simulink library "Satellite_Dynamics_lib"  (R2018b)
settings: Solver=ode45  StartTime=0.0  StopTime=10.0  RelTol=1e-3  EnableMultiTasking=on
undefined symbols (not defined in the file or in its folder): simParams
libraries: dspinverses x1, vrlib x1
settings Model: Creator=devantormey  LastModifiedBy=devantormey
settings DataIOCC: LimitDataPoints=on
settings OptimizationCC: LifeSpan=inf
settings DebuggingCC: AllowSymbolicDim=off  SFUnexpectedBacktrackingDiag=warning  SFNoUnconditionalDefaultTransitionDiag=warning
settings SFSimCC: SimUseLocalCustomCode=off
settings RTWCC: RTWUseLocalCustomCode=off
settings CodeAppCC: StateflowObjectComments=on
settings GRTTargetCC: TargetLangStandard=C89/C90 (ANSI)  GeneratePreprocessorConditionals=Disable all
settings ConfigComp: CovMetricSettings=dw  CovHtmlReporting=on  CovSaveCumulativeToWorkspaceVar=on  CovSaveSingleToWorkspaceVar=on  CovExternalEMLEnable=off

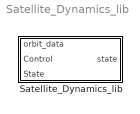
== system Satellite_Dynamics_lib ==
  Satellite_Dynamics_lib : Subsystem

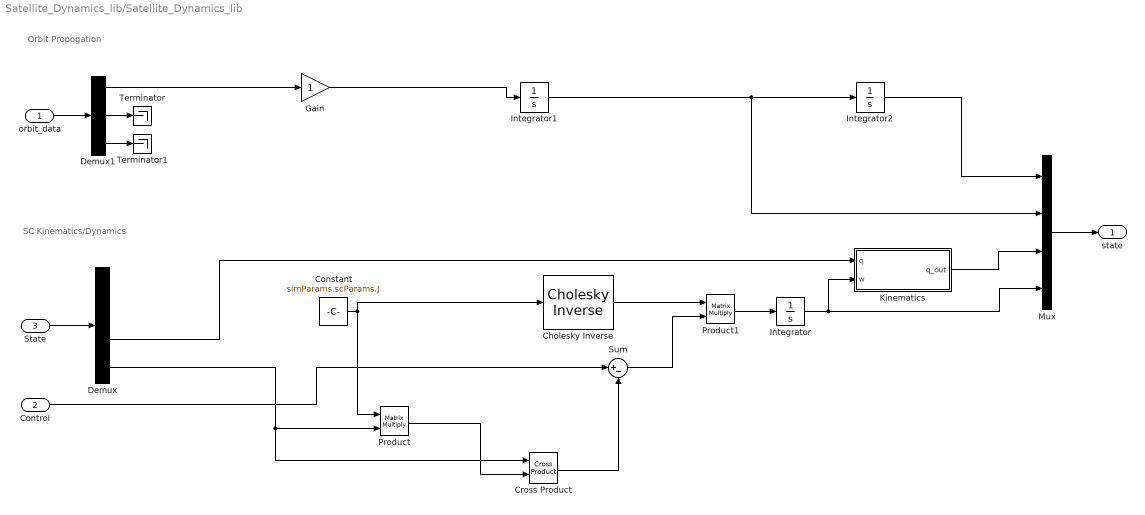
== system Satellite_Dynamics_lib/Satellite_Dynamics_lib ==
  note: Orbit Propogation
  note: SC Kinematics/Dynamics
  orbit_data : Inport
  Control : Inport  Port=2
  State : Inport  Port=3
  Cholesky Inverse : dspinverses/Cholesky Inverse  errmode=Warning
      settings: SourceProductName=DSP System Toolbox  SourceProductBaseCode=DS
  Constant : Constant  Value=simParams.scParams.J
  Cross Product : vrlib/Utilities/Cross Product
      settings: SourceProductBaseCode=VR
  Demux : Demux  Outputs=[3 3 4 3]
  Demux1 : Demux  Outputs=[3 3 1]
  Gain : Gain
  Integrator : Integrator  InitialCondition=simParams.initialConditions.w0
  Integrator1 : Integrator  InitialCondition=simParams.initialConditions.v0
  Integrator2 : Integrator  InitialCondition=simParams.initialConditions.r0
  Kinematics : Subsystem
  Mux : Mux  Inputs=[3 3 4 3]
  Product : Product  Multiplication=Matrix(*)
  Product1 : Product  Multiplication=Matrix(*)
  Sum : Sum  Inputs=|+-
  Terminator : Terminator
  Terminator1 : Terminator
  state : Outport
  wires:
  State/1 -> Demux/1
  Constant/1 -> Product/1, Cholesky Inverse/1
  Product/1 -> Cross Product/2
  Control/1 -> Sum/1
  Cross Product/1 -> Sum/2
  Sum/1 -> Product1/2
  Cholesky Inverse/1 -> Product1/1
  Product1/1 -> Integrator/1
  Integrator/1 -> Mux/4, Kinematics/2(w)
  Kinematics/1(q_out) -> Mux/3
  Mux/1 -> state/1
  Demux/3 -> Kinematics/1(q)
  Demux/4 -> Product/2, Cross Product/1
  orbit_data/1 -> Demux1/1
  Integrator1/1 -> Mux/2, Integrator2/1
  Integrator2/1 -> Mux/1
  Demux1/2 -> Terminator/1
  Demux1/3 -> Terminator1/1
  Gain/1 -> Integrator1/1
  Demux1/1 -> Gain/1

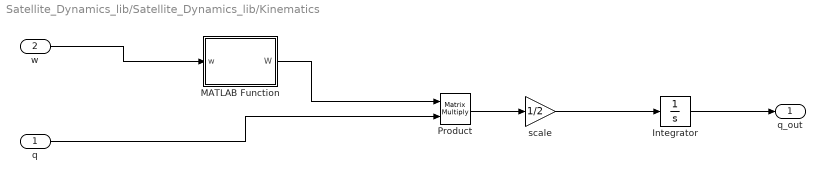
== system Satellite_Dynamics_lib/Satellite_Dynamics_lib/Kinematics ==
  q : Inport
  w : Inport  Port=2
  Integrator : Integrator  InitialCondition=simParams.initialConditions.q0
  MATLAB Function : MATLAB Function  TreatAsAtomicUnit=on
  Product : Product  Multiplication=Matrix(*)
  scale : Gain  Gain=1/2
  q_out : Outport
  wires:
  w/1 -> MATLAB Function/1(w)
  MATLAB Function/1(W) -> Product/1
  q/1 -> Product/2
  Product/1 -> scale/1
  scale/1 -> Integrator/1
  Integrator/1 -> q_out/1

== matlab function Satellite_Dynamics_lib/Kinematics/MATLAB Function ==
  data: w input; W output
function W = fcn(w)
%#codegen

W = [0, -w(1),-w(2),-w(3); w(1), 0,w(3), -w(2); w(2), -w(3), 0, w(1); w(3), w(2), -w(1), 0 ];

end
